simulink model "P2_LC"  (R2022b)
settings: Solver=VariableStepAuto  StartTime=0.0  StopTime=10.0  RelTol=1e-3
settings Model: Creator=laura  LastModifiedBy=laura

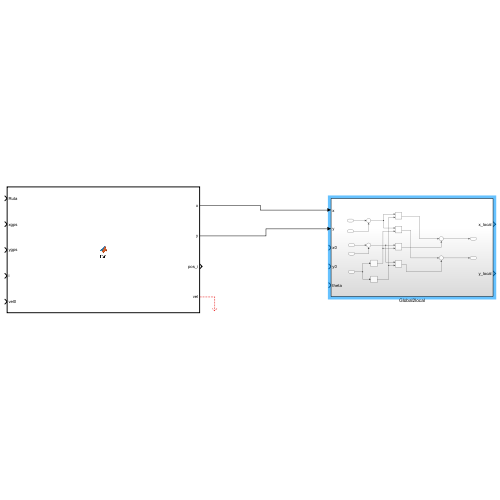
[thumbnail: Simulink's stored preview of the top-level diagram]
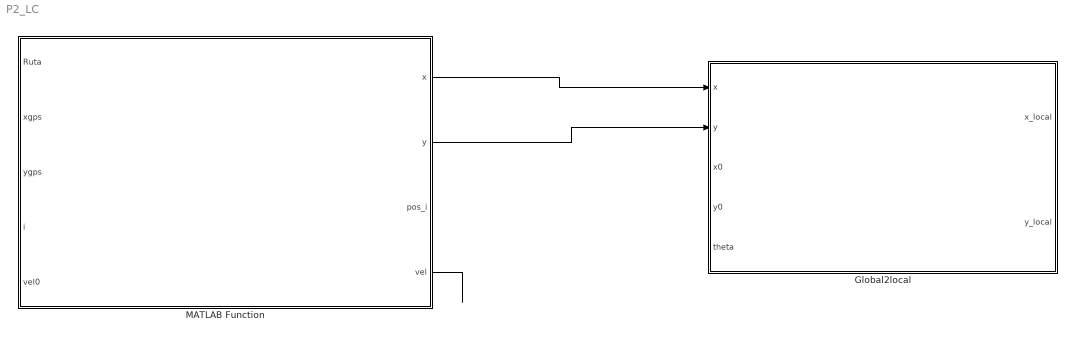
== system P2_LC ==
  Global2local : Subsystem
  MATLAB Function : MATLAB Function  TreatAsAtomicUnit=on
  wires:
  MATLAB Function/4(vel) -> ?
  MATLAB Function/1(x) -> Global2local/1(x)
  MATLAB Function/2(y) -> Global2local/2(y)

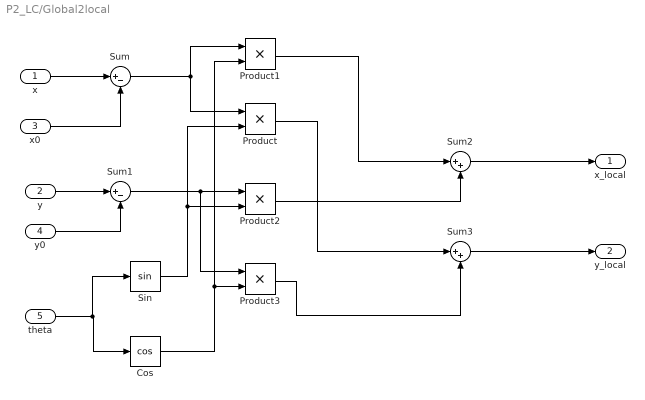
== system P2_LC/Global2local ==
  x : Inport
  y : Inport  Port=2
  x0 : Inport  Port=3
  y0 : Inport  Port=4
  theta : Inport  Port=5
  Cos : Trigonometry  Operator=cos
  Product{,1..3} (4 alike) : Product
  Sin : Trigonometry
  Sum : Sum  Inputs=|+-
  Sum1 : Sum  Inputs=|+-
  Sum2 : Sum  Inputs=|++
  Sum3 : Sum  Inputs=|++
  x_local : Outport
  y_local : Outport  Port=2
  wires:
  x/1 -> Sum/1
  y0/1 -> Sum1/2
  y/1 -> Sum1/1
  x0/1 -> Sum/2
  theta/1 -> Sin/1, Cos/1
  Cos/1 -> Product3/2, Product1/2
  Sum/1 -> Product/1, Product1/1
  Sin/1 -> Product2/2, Product/2
  Sum1/1 -> Product3/1, Product2/1
  Product1/1 -> Sum2/1
  Product2/1 -> Sum2/2
  Product/1 -> Sum3/1
  Product3/1 -> Sum3/2
  Sum3/1 -> y_local/1
  Sum2/1 -> x_local/1

== matlab function P2_LC/MATLAB Function ==
  data: x output; Ruta input; y output; xgps input; ygps input; i input; vel0 input; pos_i output; vel output
function [x,y,pos_i,vel] = fcn(Ruta,xgps,ygps,i,vel0)
%Seleccionamos punto objetivo
pos_i=i;
%Obtener puntos ruta 
[fila,~]= size(Ruta);
%Distancia entre punto objetivo y pos_act 
xdif=Ruta((pos_i+1),1)-xgps;
ydif=Ruta((pos_i+1),2)-ygps;
%Calculamos el modulo
mod=sqrt(xdif^2+ydif^2);
%Mantenemos velocidad
vel=vel0;

if mod<1
    pos_i=pos_i+1;
    vel=1.2;
end
if pos_i+1>fila
    vel=0;
end

x=Ruta((pos_i+1),1);
y=Ruta((pos_i+1),2);
end
